simulink model "singulardelay"  (R2016b)
settings: Solver=ode45  StartTime=0.0  StopTime=15  RelTol=1e-3  EnableMultiTasking=on
values from neighbouring files (symbols this model uses):
  B = [0 0 0 1]    [singular.mat]
  f = F'    [resposta_no_tempo.m]    (also in singular.mat = [4.07498079774 -6.5522232211 -2.04658222993 -4.85411624646])
  g = G'    [resposta_no_tempo.m]    (also in singular.mat = [-8.72247241851 4.87703707426 1.84253176904 -2.73047545799])
  tau = 0.1    [singular.mat]
libraries: cstblocks x1
settings Model: Creator=profj  LastModifiedBy=danta
settings DataIOCC: LimitDataPoints=on  SaveFormat=Array
settings OptimizationCC: LifeSpan=inf
settings DebuggingCC: SFUnexpectedBacktrackingDiag=warning  SFNoUnconditionalDefaultTransitionDiag=warning  SFExecutionAtInitializationDiag=none
settings HardwareCC: ProdBitPerPointer=32  ProdBitPerSizeT=32  ProdBitPerPtrDiffT=32  ProdLargestAtomicFloat=None  ProdIntDivRoundTo=Undefined  ProdEndianess=Unspecified  ProdWordSize=32  ProdHWDeviceType=32-bit Generic
settings ModelReferenceCC: PropagateSignalLabelsOutOfModel=off
settings GRTTargetCC: TargetLangStandard=C89/C90 (ANSI)  GeneratePreprocessorConditionals=Disable all
settings ConfigComp: CovMetricSettings=dw  CovHtmlReporting=on  CovSaveCumulativeToWorkspaceVar=on  CovSaveSingleToWorkspaceVar=on  CovExternalEMLEnable=off

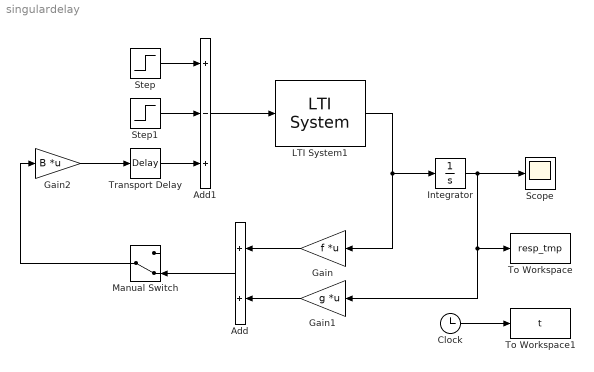
== system singulardelay ==
  Add : Sum
  Add1 : Sum  Inputs=+-+
  Clock : Clock
  Gain : Gain  Gain=f  Multiplication=Matrix(K*u)
  Gain1 : Gain  Gain=g  Multiplication=Matrix(K*u)
  Gain2 : Gain  Gain=B  Multiplication=Matrix(K*u)
  Integrator : Integrator
  LTI System1 : cstblocks/LTI System  sys=Hs  IC=[]
  Manual Switch : ManualSwitch  CurrentSetting=0
  Scope : Scope
  Step : Step  Time=0  After=5  SampleTime=0
  Step1 : Step  After=5  SampleTime=0
  To Workspace : ToWorkspace  VariableName=resp_tmp  SampleTime=-1
  To Workspace1 : ToWorkspace  VariableName=t  SampleTime=-1
  Transport Delay : TransportDelay  DelayTime=tau
  wires:
  LTI System1/1 -> Gain/1, Integrator/1
  Integrator/1 -> Scope/1, To Workspace/1, Gain1/1
  Gain/1 -> Add/1
  Gain1/1 -> Add/2
  Gain2/1 -> Transport Delay/1
  Add1/1 -> LTI System1/1
  Add/1 -> Manual Switch/2
  Manual Switch/1 -> Gain2/1
  Step/1 -> Add1/1
  Transport Delay/1 -> Add1/3
  Step1/1 -> Add1/2
  Clock/1 -> To Workspace1/1
